simulink model "GMSK_PLL_Tx"  (R2024a)
settings: Solver=VariableStepAuto  StartTime=0.0  StopTime=4e-5  FixedStep=DESIGN_CONST.Tsim  RelTol=1e-3
model workspace (MAT data in the model file):
  Frequency_78 = 900000016.03
  Frequency_93 = 799999936
  TargetFrequency_78 = 900000000
  TargetFrequency_93 = 900000000
  uniqueStringPll_37 = '91_5736'
  uniqueStringPll_78 = '17_1187'
  uniqueStringPll_93 = '90_5792'
  uniqueString_93 = '81_4724'
undefined symbols (not defined in the file or in its folder): DESIGN_CONST, fdesignblkfcn, gcbh
libraries: msbPllFoundation x4, simulink_extras x3, dspsigops x1, dsparch4 x1
settings Model: Creator=Sayantan  LastModifiedBy=Sayantan

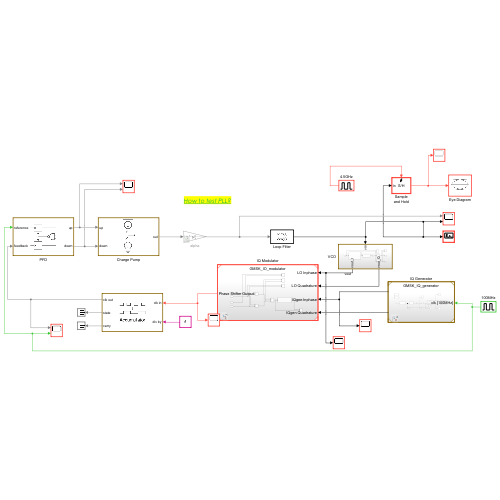
[thumbnail: Simulink's stored preview of the top-level diagram]
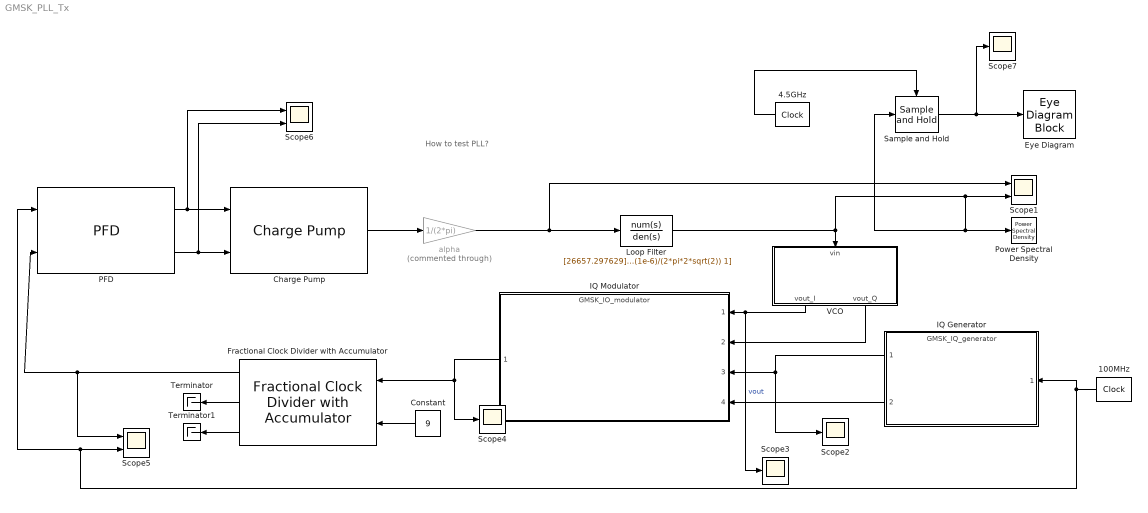
== system GMSK_PLL_Tx ==
  note: How to test PLL?
  100MHz : simulink_extras/Flip Flops/Clock  period=DESIGN_CONST.T
  4.5GHz : simulink_extras/Flip Flops/Clock  period=DESIGN_CONST.Tsim*2
  Charge Pump : msbPllFoundation/Charge Pump  OutputCurrent=100e-6  InputThreshold=0.5  ExtraBuffer=off  NBuffer=1000  EnableCurrentImpairments=off  CurrentImbalance=1e-7  LeakageCurrent=1e-8  EnableTimingImpairments=off  DefaultOrAdvanced=Default  MaxFreqInterest=10e9  RiseFallUp=5e-9  PropDelayUp=6e-9  RiseFallDown=2e-9  PropDelayDown=4e-9
  Constant : Constant  Value=9
  Eye Diagram : EyeDiagramBlock  WindowPosition=[0.000000,12.000000,1366.000000,745.000000,]  ScopeFrameLocation=window  SamplesPerSymbol=100  SampleOffset=100  YLimits=[-0.07771550120080506,0.0870850616659638]  PlotImaginaryAxes=off
  Fractional Clock Divider with Accumulator : msbPllFoundation/Fractional Clock Divider with Accumulator  ExtraBuffer=off  NBuffer=1000
  IQ Generator : ModelReference  ModelNameDialog=GMSK_IQ_generator.slx  SimulationMode=Normal  ModelReferenceVersion=1.48
  IQ Modulator : ModelReference  ModelNameDialog=GMSK_IO_modulator.slx  SimulationMode=Normal  ModelReferenceVersion=1.13
  Loop Filter : TransferFcn  Numerator=[26657.297629]  Denominator=[(1e-6)/(2*pi*2*sqrt(2)) 1]
  PFD : msbPllFoundation/PFD  DeadbandCompensation=30e-12  ExtraBuffer=off  NBuffer=1000  EnableImpairments=off  DefaultOrAdvanced=Default  MaxFreqInterest=10e9  RiseFallTime=30e-12  PropDelay=50e-12
  Power Spectral Density : simulink_extras/Additional Sinks/Power Spectral Density  npts=10240  fftpts=1024  HowOften=1024  sampleT=DESIGN_CONST.Tsim
  Sample and Hold : dspsigops/Sample and Hold  trig=Rising edge  initCond=0  latchinput=off
  Scope1 : Scope  NumInputPorts=2
  Scope{2..4,7} (4 alike) : Scope
  Scope5 : Scope  NumInputPorts=2
  Scope6 : Scope  NumInputPorts=2
  Terminator : Terminator
  Terminator1 : Terminator
  VCO : Subsystem
  alpha : Gain  Commented=through  Gain=1/(2*pi)
  wires:
  PFD/1 -> Scope6/1, Charge Pump/1
  PFD/2 -> Scope6/2, Charge Pump/2
  Charge Pump/1 -> alpha/1
  alpha/1 -> Scope1/1, Loop Filter/1
  VCO/1(vout_I) -> Scope3/1, IQ Modulator/1  "vout"
  Loop Filter/1 -> Sample and Hold/1, Power Spectral Density/1, Scope1/2, VCO/1(vin)
  IQ Modulator/1 -> Fractional Clock Divider with Accumulator/1, Scope4/1
  100MHz/1 -> PFD/1, Scope5/2, IQ Generator/1
  VCO/2(vout_Q) -> IQ Modulator/2
  IQ Generator/1 -> Scope2/1, IQ Modulator/3
  IQ Generator/2 -> IQ Modulator/4
  Sample and Hold/1 -> Scope7/1, Eye Diagram/1
  4.5GHz/1 -> Sample and Hold/Trigger
  Fractional Clock Divider with Accumulator/1 -> Scope5/1, PFD/2
  Constant/1 -> Fractional Clock Divider with Accumulator/2
  Fractional Clock Divider with Accumulator/2 -> Terminator/1
  Fractional Clock Divider with Accumulator/3 -> Terminator1/1

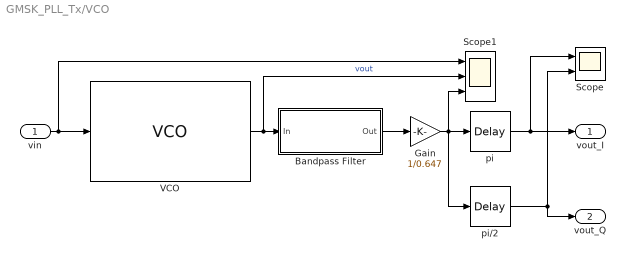
== system GMSK_PLL_Tx/VCO ==
  vin : Inport
  Bandpass Filter : Subsystem  DialogController=fdesignblkfcn  InitFcn=fdesignblkfcn(gcbh, {'InitFcn'});  mask(Bandpass Filter){}
      mask help: dsp:DSPFilterDesignBlockDialog:BandpassFdesign_MaskDesc
      settings: CopyFcn=fdesignblkfcn(gcbh, {'CopyFcn'});
      mask Help: helpview(mapfilelocation('dsp'), 'dspbandpassfilter');
      mask Display: disp('Bandpass');
  Gain : Gain  Gain=1/0.647
  Scope : Scope  NumInputPorts=2
  Scope1 : Scope  NumInputPorts=3
  VCO : msbPllFoundation/VCO  SpecifyUsing=Voltage sensitivity  Kvco=30e6  Fo=900e6  ControlVoltage=[-5 0 5]  OutputFrequency=[2e9 2.5e9 3e9]  Amplitude=1  ExtraBuffer=off  NBuffer=1000  AddPhaseNoise=off  Foffset=[10e3 100e3 1e6 3e6 10e6]  PhaseNoise=[-77 -108 -134 -145 -154]  MaxKvco=30000000
  pi : TransportDelay  DelayTime=2/(4*900e6)
  pi/2 : TransportDelay  DelayTime=1/(4*900e6)
  vout_I : Outport
  vout_Q : Outport  Port=2
  wires:
  vin/1 -> Scope1/1, VCO/1
  VCO/1 -> Bandpass Filter/1(In), Scope1/2  "vout"
  Bandpass Filter/1(Out) -> Gain/1
  pi/1 -> Scope/1, vout_I/1
  Gain/1 -> Scope1/3, pi/2/1, pi/1
  pi/2/1 -> vout_Q/1, Scope/2

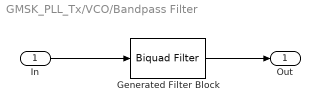
== system GMSK_PLL_Tx/VCO/Bandpass Filter ==
  In : Inport
  Generated Filter Block : dsparch4/Biquad Filter  Tag=BlockMethodSubSystem  FilterSource=Dialog parameters  CoeffSource=Specify via dialog  FilterObject=BQF  IIRFiltStruct=Direct form II  BiQuadCoeffs=[0.0149727657479659469 0 -0.0149727657479659469 1 -1.61490323215326148 0.985448277219509006;0.0102162091169220107 0 -0.0102162091169220107 1 -1.59738013834248438 0.98515077162607656;0.0105376594927481162 0 -0.0105376594927481162 1 -1.6034961418583582 0.979570694823028054;0.00412973010843779333 0 -0.00412973010843779333 1 -1.59960968370924173 0.979479275997838683;0.02039774232704792 0 -0.02039774232704792 1 -1.62748044297368111 0.996775722269118702;0.0102786313885339219 0 -0.0102786313885339219 1 -1.60312741008854576 0.996682745258407721;0.0135889301744539729 0 -0.0135889301744539729 1 -1.6087627076574913 0.981630965044335335;0.00575487462043394651 0 -0.00575487462043394651 1 -1.59749352823360824 0.981391165564786894;0.0186939700284457742 0 -0.0186939700284457742 1 -1.62134189328779765 0.990658082995132583;0.859059466175205566 0 -0.859059466175205566 1 -1.59931232438214455 0.990416154652342673]  ScaleValues=[0.00846546727472092739;1;1;1;1;1;1;1;1;1;1]  IC=0  ICnum=0  ICden=0  a0Flag=Warning  optimizeScaleValues=off  ScaleValueMode=Specify via input port (g)  InputProcessing=Columns as channels (frame based)  roundingMode=Floor  overflowMode=off  scaleValueFracLength=14  denProdOutputFracLength=30  denAccumFracLength=30  secondMemoryFracLength=15
  Out : Outport  VectorParamsAs1DForOutWhenUnconnected=off
  wires:
  In/1 -> Generated Filter Block/1
  Generated Filter Block/1 -> Out/1
